simulink model "real_plant_A_2013B"  (R2013b)
settings: Solver=ode1  StartTime=0.0  StopTime=sim_run  FixedStep=0.001  RelTol=1e-3
undefined symbols (not defined in the file): AD622, Humusoft, Serial_Port, Standard_Devices, UDP_Protocol, zh_step
libraries: rtwinlib x4
settings Model: CovModelRefEnable=off  Creator=Anony  LastModifiedBy=dave
settings DataIOCC: SaveFormat=StructureWithTime
settings DebuggingCC: UnderspecifiedInitializationDetection=Simplified  MergeDetectMultiDrivingBlocksExec=error  SolverPrmCheckMsg=none  FrameProcessingCompatibilityMsg=error
settings HardwareCC: ProdBitPerPointer=64  ProdLargestAtomicFloat=Float  ProdIntDivRoundTo=Zero  ProdEndianess=LittleEndian  ProdHWDeviceType=Specified
settings GRTTargetCC: CodeReplacementLibrary=C89/C90 (ANSI)  GeneratePreprocessorConditionals=Use local settings

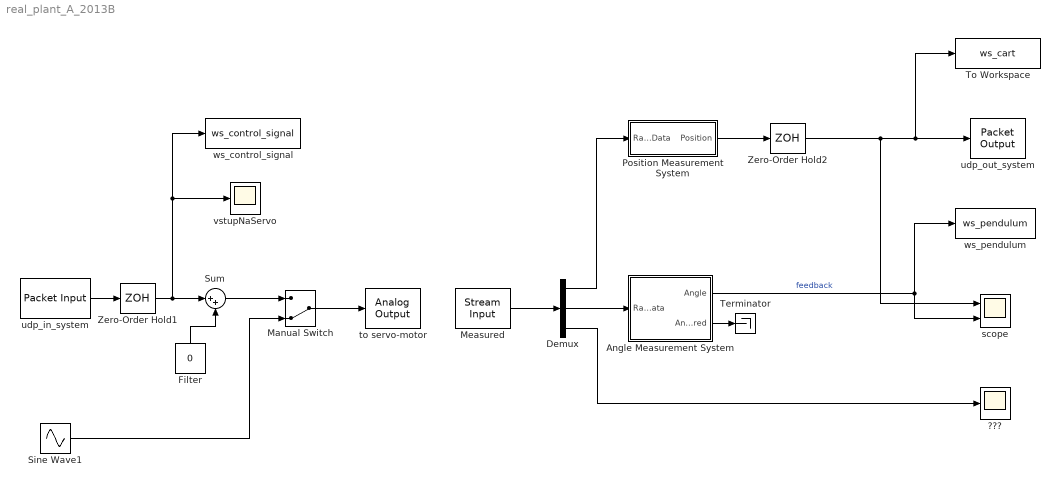
== system real_plant_A_2013B ==
  "???" : Scope
      settings: TimeRange=auto  LimitDataPoints=on  MaxDataPoints=5000  SaveToWorkspace=off  SaveName=ScopeData2  YMin=1945.6  YMax=2150.4  SampleTime=-1
  Angle Measurement System : Subsystem
  Demux : Demux  Outputs=3
  "Filter " : Constant  Value=0
  Manual Switch : ManualSwitch  CurrentSetting=0
  Measured : rtwinlib/Stream Input  SampleTime=0.001  MaxMissedTicks=inf  ShowMissedTicks=off  YieldWhenWaiting=off  DrvName=Standard_Devices/Serial_Port  DrvAddress=1  DrvOptions=[115200 8 0 0 0 0 0 1]  DataTypes='3*double'  FormatString='%f%f%f'  Terminator={'\r\n'}  ShowReady=off  ShowError=off
      settings: AttributesFormatString=Standard Devices\nSerial Port [1h]
  Position Measurement System : Subsystem
  Sine Wave1 : Sin  Amplitude=4  SampleTime=0
  Sum : Sum  Inputs=|++
  Terminator : Terminator
  To Workspace : ToWorkspace  VariableName=ws_cart  SaveFormat=Timeseries  SampleTime=-1
  Zero-Order Hold1 : ZeroOrderHold  SampleTime=zh_step
  Zero-Order Hold2 : ZeroOrderHold  SampleTime=zh_step
  scope : Scope  NumInputPorts=2
      settings: TimeRange=auto  MaxDataPoints=5000  SaveToWorkspace=off  YMin=-1.00000~15.00000  YMax=1.00000~35.00000  SampleTime=-1
  to servo-motor : rtwinlib/Analog Output  SampleTime=0.001  MaxMissedTicks=inf  ShowMissedTicks=off  YieldWhenWaiting=off  DrvName=Humusoft/AD622  DrvAddress=4294967295  DrvOptions=zeros(1,0)  Channels=2  RangeMode=1  VoltRange=1  InitialValue=0  FinalValue=0
      settings: AttributesFormatString=Humusoft\nAD622 [auto]
  udp_in_system : rtwinlib/Packet Input  SampleTime=0.001  MaxMissedTicks=inf  ShowMissedTicks=off  YieldWhenWaiting=off  DrvName=Standard_Devices/UDP_Protocol  DrvAddress=20500  DrvOptions=[2468394756 20500]  PacketSize=8  DataTypes='double'  ShowReady=off  ShowError=off  PacketID=1  ByteOrder=1  ShowTimestamp=off
  udp_out_system : rtwinlib/Packet Output  SampleTime=0.01  MaxMissedTicks=inf  ShowMissedTicks=off  YieldWhenWaiting=off  DrvName=Standard_Devices/UDP_Protocol  DrvAddress=21500  DrvOptions=[2468394756 21500]  PacketSize=8  DataTypes='double'  ShowReady=off  ShowError=off  PacketID=1  ByteOrder=1  InitialValue=[]  FinalValue=[]
  vstupNaServo : Scope
      settings: TimeRange=10  MaxDataPoints=5000  SaveName=ScopeData  YMin=-1.00000  YMax=1.00000  SampleTime=-1
  ws_control_signal : ToWorkspace  VariableName=ws_control_signal  SaveFormat=Timeseries  SampleTime=-1
  ws_pendulum : ToWorkspace  VariableName=ws_pendulum  SaveFormat=Timeseries  SampleTime=-1
  wires:
  Zero-Order Hold1/1 -> Sum/1, ws_control_signal/1, vstupNaServo/1
  udp_in_system/1 -> Zero-Order Hold1/1
  Measured/1 -> Demux/1
  Angle Measurement System/1(Angle) -> ws_pendulum/1, scope/2  "feedback"
  Zero-Order Hold2/1 -> scope/1, To Workspace/1, udp_out_system/1
  Angle Measurement System/2(Angle Filtered) -> Terminator/1
  Demux/1 -> Position Measurement System/1(Raw Data)
  Position Measurement System/1(Position) -> Zero-Order Hold2/1
  Demux/2 -> Angle Measurement System/1(RawData)
  Demux/3 -> "???"/1
  "Filter "/1 -> Sum/2
  Sine Wave1/1 -> Manual Switch/2
  Sum/1 -> Manual Switch/1
  Manual Switch/1 -> to servo-motor/1

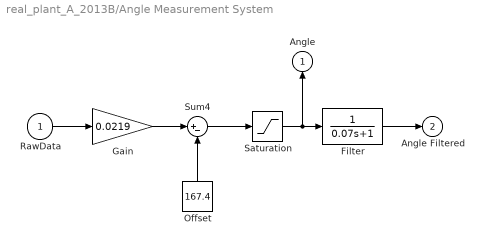
== system real_plant_A_2013B/Angle Measurement System ==
  RawData : Inport
  Filter : TransferFcn  Denominator=[0.07 1]
  Gain : Gain  Gain=0.0219
  Offset : Constant  Value=167.4
  Saturation : Saturate  UpperLimit=90  LowerLimit=-90
  Sum4 : Sum  Inputs=|+-
  Angle : Outport
  Angle Filtered : Outport  Port=2
  wires:
  RawData/1 -> Gain/1
  Offset/1 -> Sum4/2
  Sum4/1 -> Saturation/1
  Gain/1 -> Sum4/1
  Filter/1 -> Angle Filtered/1
  Saturation/1 -> Filter/1, Angle/1

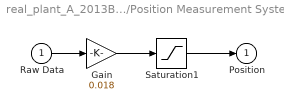
== system real_plant_A_2013B/Position Measurement System ==
  Raw Data : Inport
  Gain : Gain  Gain=0.018
  Saturation1 : Saturate  UpperLimit=1600  LowerLimit=0
  Position : Outport
  wires:
  Gain/1 -> Saturation1/1
  Saturation1/1 -> Position/1
  Raw Data/1 -> Gain/1
